simulink model "Simulink_B_8_5"  (R2017b)
settings: Solver=VariableStepAuto  StartTime=0.0  StopTime=10.0  RelTol=1e-3
settings Model: Creator=LUCIA  LastModifiedBy=LUCIA

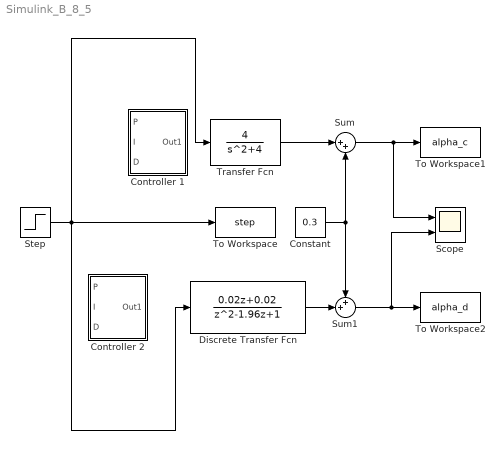
== system Simulink_B_8_5 ==
  Constant : Constant  Value=0.3
  Controller 1 : Subsystem
  Controller 2 : Subsystem
  Discrete Transfer Fcn : DiscreteTransferFcn  Numerator=[0.02 0.02]  Denominator=[1 -1.96 1]  SampleTime=0.1
  Scope : Scope  NumInputPorts=2
  Step : Step  After=8  SampleTime=0
  Sum : Sum  Inputs=|++
  Sum1 : Sum  Inputs=++|
  To Workspace : ToWorkspace  VariableName=step  SaveFormat=Timeseries  SampleTime=-1
  To Workspace1 : ToWorkspace  VariableName=alpha_c  SaveFormat=Timeseries  SampleTime=-1
  To Workspace2 : ToWorkspace  VariableName=alpha_d  SaveFormat=Timeseries  SampleTime=-1
  Transfer Fcn : TransferFcn  Numerator=4  Denominator=[1 0 4]
  wires:
  Transfer Fcn/1 -> Sum/1
  Constant/1 -> Sum1/1, Sum/2
  Discrete Transfer Fcn/1 -> Sum1/2
  Step/1 -> To Workspace/1, Transfer Fcn/1, Discrete Transfer Fcn/1
  Sum1/1 -> Scope/2, To Workspace2/1
  Sum/1 -> Scope/1, To Workspace1/1

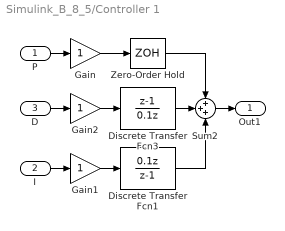
== system Simulink_B_8_5/Controller 1 ==
  P : Inport
  "I " : Inport  Port=2
  D : Inport  Port=3
  Discrete Transfer Fcn1 : DiscreteTransferFcn  Numerator=[0.1 0]  Denominator=[1 -1]  SampleTime=0.1
  Discrete Transfer Fcn3 : DiscreteTransferFcn  Numerator=[1 -1]  Denominator=[0.1 0]  SampleTime=0.1
  Gain : Gain
  Gain1 : Gain
  Gain2 : Gain
  Sum2 : Sum  Inputs=+++
  Zero-Order Hold : ZeroOrderHold  SampleTime=-1
  Out1 : Outport
  wires:
  Discrete Transfer Fcn3/1 -> Sum2/2
  Gain2/1 -> Discrete Transfer Fcn3/1
  Gain1/1 -> Discrete Transfer Fcn1/1
  Zero-Order Hold/1 -> Sum2/1
  Discrete Transfer Fcn1/1 -> Sum2/3
  Gain/1 -> Zero-Order Hold/1
  D/1 -> Gain2/1
  P/1 -> Gain/1
  Sum2/1 -> Out1/1
  "I "/1 -> Gain1/1

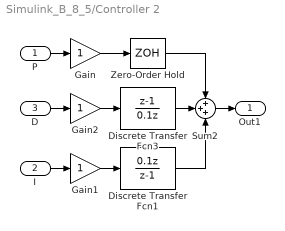
== system Simulink_B_8_5/Controller 2 ==
  P : Inport
  "I " : Inport  Port=2
  D : Inport  Port=3
  Discrete Transfer Fcn1 : DiscreteTransferFcn  Numerator=[0.1 0]  Denominator=[1 -1]  SampleTime=0.1
  Discrete Transfer Fcn3 : DiscreteTransferFcn  Numerator=[1 -1]  Denominator=[0.1 0]  SampleTime=0.1
  Gain : Gain
  Gain1 : Gain
  Gain2 : Gain
  Sum2 : Sum  Inputs=+++
  Zero-Order Hold : ZeroOrderHold  SampleTime=-1
  Out1 : Outport
  wires:
  Discrete Transfer Fcn3/1 -> Sum2/2
  Gain2/1 -> Discrete Transfer Fcn3/1
  Gain1/1 -> Discrete Transfer Fcn1/1
  Zero-Order Hold/1 -> Sum2/1
  Discrete Transfer Fcn1/1 -> Sum2/3
  Gain/1 -> Zero-Order Hold/1
  D/1 -> Gain2/1
  P/1 -> Gain/1
  Sum2/1 -> Out1/1
  "I "/1 -> Gain1/1
